simulink model "Joystick_Visualization_2019a"  (R2019a)
settings: Solver=ode1  StartTime=0.0  StopTime=inf  FixedStep=0.001  RelTol=1e-3  EnableMultiTasking=on
undefined symbols (not defined in the file): Host, Visualization
libraries: quarc_library x25, simulink x5
settings Model: SimulationMode=external  ExtModeTrigDuration=10000  Creator=Admin  LastModifiedBy=lgonzalez
settings SolverCC: PositivePriorityOrder=on
settings DataIOCC: SaveFormat=StructureWithTime  ReturnWorkspaceOutputs=off
settings DebuggingCC: SFUnexpectedBacktrackingDiag=warning  SFNoUnconditionalDefaultTransitionDiag=warning  SFExecutionAtInitializationDiag=none  ArithmeticOperatorsInVariantConditions=warning
settings SFSimCC: SimUseLocalCustomCode=off
settings RTWCC: Description=QUARC Win64 Target Using Toolchain  SystemTargetFile=quarc_win64.tlc  TemplateMakefile=quarc_default_tmf  RTWUseLocalCustomCode=off  Toolchain=QUARC win64 | nmake (64-bit Windows)  BuildConfiguration=Faster Runs
settings CodeAppCC: StateflowObjectComments=on
settings STFCustomTargetCC: ConcurrentExecutionCompliant=on  UseToolchainInfoCompliant=on  SystemTargetFile=quarc_win64.tlc
settings GRTTargetCC: TargetLangStandard=C89/C90 (ANSI)  ParMdlRefBuildCompliant=off  CompOptLevelCompliant=off  CombineOutputUpdateFcns=off  MatFileLogging=off  CPPClassGenCompliant=off  GRTInterface=on  ExtMode=on  ExtModeMexFile=quarc_comm
settings ConfigComp: CovMetricSettings=dw  CovSaveCumulativeToWorkspaceVar=on  CovSaveSingleToWorkspaceVar=on  CovExternalEMLEnable=off

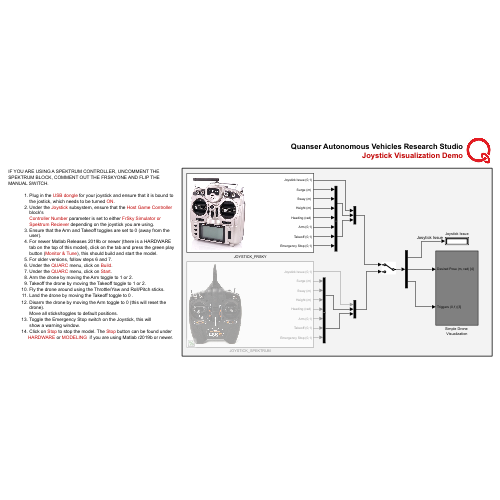
[thumbnail: Simulink's stored preview of the top-level diagram]
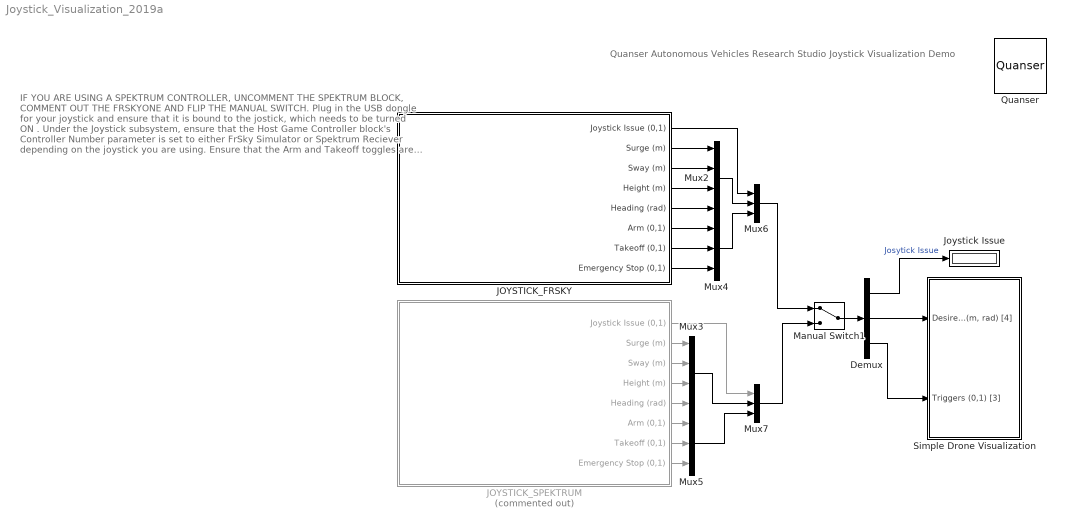
== system Joystick_Visualization_2019a ==
  note: IF YOU ARE USING A SPEKTRUM CONTROLLER, UNCOMMENT THE SPEKTRUM BLOCK, COMMENT OUT THE FRSKYONE AND FLIP THE MANUAL SWITCH.
      |
      | Plug in the USB dongle for your joystick and ensure that it is bound to the jostick, which needs to be turned ON .
      | Under the Joystick subsystem, ensure that the Host Game Controller block's
      | Controller Number parameter is set to either FrSky Simulator or Spektrum Reciever depending on the joystick you are using.
      | Ensure that the Arm and Takeoff toggles are set to 0 (away from the user).
      | For newer Matlab Releases 2019b or newer (there is a HARDWARE tab on the top of this model), click on the tab and press the green play button ( Monitor & Tune ), this should build and start the model.
      | For older versions, follow steps 6 and 7.
      | Under the QUARC menu, click on Build .
      | Under the QUARC menu, click on Start .
      | Arm the drone by moving the Arm toggle to 1 or 2.
      | Takeoff the drone by moving the Takeoff toggle to 1 or 2.
      | Fly the drone around using the Throttle/Yaw and Roll/Pitch sticks.
      | Land the drone by moving the Takeoff toggle to 0 .
      | Disarm the drone by moving the Arm toggle to 0 (this will reset the drone).
      | Move all sticks/toggles to default positions.
      | Toggle the Emergency Stop switch on the Joystick, this will
      | show a warning window.
      | Click on Stop to stop the model. The Stop button can be found under
      | HARDWARE or MODELING if you are using Matlab r2019b or newer.
  note: Quanser Autonomous Vehicles Research Studio
      | Joystick Visualization Demo
  Demux : Demux  Outputs=[1 4 3]
  JOYSTICK_FRSKY : Subsystem
      mask Display: image('frsky.jpg')
  JOYSTICK_SPEKTRUM : Subsystem  Commented=on
      mask Display: image('spektrum.jpg')
  Joystick Issue : Display
      settings: Decimation=400
  Manual Switch1 : ManualSwitch
  Mux2 : Mux
  Mux3 : Mux
  Mux{4..7} (4 alike) : Mux  Inputs=3
  Quanser : quarc_library/Logos/Quanser
  Simple Drone Visualization : Subsystem
  wires:
  Demux/2 -> Simple Drone Visualization/1("Desired Pose (m, rad) [4]")
  Demux/3 -> Simple Drone Visualization/2(Triggers (0,1) [3])
  JOYSTICK_FRSKY/2("Surge (m) ") -> Mux2/1
  JOYSTICK_FRSKY/3("Sway (m) ") -> Mux2/2
  JOYSTICK_FRSKY/4("Height (m) ") -> Mux2/3
  JOYSTICK_FRSKY/5("Heading (rad) ") -> Mux2/4
  JOYSTICK_FRSKY/8(Emergency Stop (0,1)) -> Mux4/3
  JOYSTICK_FRSKY/7(Takeoff (0,1)) -> Mux4/2
  JOYSTICK_FRSKY/6(Arm (0,1)) -> Mux4/1
  JOYSTICK_SPEKTRUM/6(Arm (0,1)) -> Mux5/1
  JOYSTICK_SPEKTRUM/7(Takeoff (0,1)) -> Mux5/2
  JOYSTICK_SPEKTRUM/8(Emergency Stop (0,1)) -> Mux5/3
  JOYSTICK_SPEKTRUM/2("Surge (m) ") -> Mux3/1
  JOYSTICK_SPEKTRUM/3("Sway (m) ") -> Mux3/2
  JOYSTICK_SPEKTRUM/4("Height (m) ") -> Mux3/3
  JOYSTICK_SPEKTRUM/5("Heading (rad) ") -> Mux3/4
  Mux2/1 -> Mux6/2
  Mux4/1 -> Mux6/3
  Mux3/1 -> Mux7/2
  Mux5/1 -> Mux7/3
  Manual Switch1/1 -> Demux/1
  Mux6/1 -> Manual Switch1/1
  Mux7/1 -> Manual Switch1/2
  JOYSTICK_FRSKY/1(Joystick Issue (0,1)) -> Mux6/1
  JOYSTICK_SPEKTRUM/1(Joystick Issue (0,1)) -> Mux7/1
  Demux/1 -> Joystick Issue/1  "Josytick Issue"

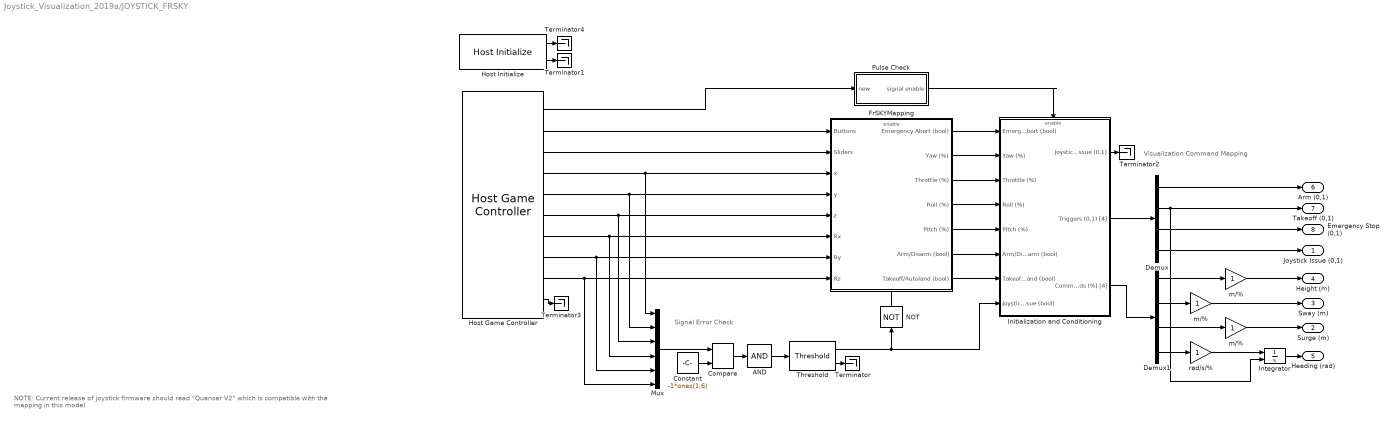
== system Joystick_Visualization_2019a/JOYSTICK_FRSKY ==
  note: NOTE: Current release of joystick firmware should read "Quanser V2" which is compatible with the mapping in this model
  note: Visualization Command Mapping
  note: Signal Error Check
  "  m/%  " : Gain
  " m/% " : Gain
  " rad/s/%" : Gain
  AND : Logic  Inputs=1  AllPortsSameDT=off  OutDataTypeStr=boolean
  Compare : quarc_library/Logic Operations/Compare  operator===  output_data_type=boolean
      settings: SourceProductName=QUARC Targets
  Constant : Constant  Value=-1*ones(1,6)
  Demux : Demux
  Demux1 : Demux
  FrSKYMapping : Subsystem
  Host Game Controller : quarc_library/Devices/Peripherals/Host/Host Game Controller  object_name=Host-1  controller=1  buffer_size=20  deadzone=[]  saturation=[]  sample_time=qc_get_step_size  auto_center=off  enabled=on  debug_mode=off
      settings: SourceProductName=QUARC Targets
  Host Initialize : quarc_library/Devices/Peripherals/Host/Host Initialize  object_name=Host-1  uri_source=Use external mode communications  uri=tcpip://localhost:18001  send_buffer_size=1000  receive_buffer_size=1000  thread_priority=0  run_client=on  use_window=off  window_position=[]  sample_time=qc_get_step_size  active=on
      settings: SourceProductName=QUARC Targets
  Initialization and Conditioning : Subsystem  TreatAsAtomicUnit=on
  Integrator : Integrator  ExternalReset=falling
  Mux : Mux  Inputs=6
  NOT : Logic  Operator=NOT  IconShape=distinctive  AllPortsSameDT=off  OutDataTypeStr=boolean
  Pulse Check : Subsystem  TreatAsAtomicUnit=on
  Terminator{,1..4} (5 alike) : Terminator
  Threshold : quarc_library/Discontinuities/Threshold  operator=>=  param_src=Specify via dialog  threshold=0.5  duration=0.2
      settings: SourceProductName=QUARC Targets
  m/% : Gain
  Joystick Issue (0,1) : Outport  VectorParamsAs1DForOutWhenUnconnected=off
  "Surge (m) " : Outport  Port=2  VectorParamsAs1DForOutWhenUnconnected=off
  "Sway (m) " : Outport  Port=3  VectorParamsAs1DForOutWhenUnconnected=off
  "Height (m) " : Outport  Port=4  VectorParamsAs1DForOutWhenUnconnected=off
  "Heading (rad) " : Outport  Port=5  VectorParamsAs1DForOutWhenUnconnected=off
  Arm (0,1) : Outport  Port=6  VectorParamsAs1DForOutWhenUnconnected=off
  Takeoff (0,1) : Outport  Port=7  VectorParamsAs1DForOutWhenUnconnected=off
  Emergency Stop (0,1) : Outport  Port=8  VectorParamsAs1DForOutWhenUnconnected=off
  wires:
  Host Initialize/1 -> Terminator4/1
  Host Initialize/2 -> Terminator1/1
  Host Game Controller/7 -> Mux/4, FrSKYMapping/6(Rx)
  Constant/1 -> Compare/2
  Threshold/2 -> Terminator/1
  Host Game Controller/10 -> Terminator3/1
  Mux/1 -> Compare/1
  FrSKYMapping/2(Yaw (%)) -> Initialization and Conditioning/2(Yaw (%))
  Host Game Controller/3 -> FrSKYMapping/2(Sliders)
  Host Game Controller/6 -> Mux/3, FrSKYMapping/5(z)
  Initialization and Conditioning/1(Joystick Issue (0,1)) -> Terminator2/1
  " m/% "/1 -> "Sway (m) "/1
  Host Game Controller/9 -> Mux/6, FrSKYMapping/8(Rz)
  FrSKYMapping/3(Throttle (%)) -> Initialization and Conditioning/3(Throttle (%))
  FrSKYMapping/4(Roll (%)) -> Initialization and Conditioning/4(Roll (%))
  Host Game Controller/4 -> Mux/1, FrSKYMapping/3(x)
  Host Game Controller/1 -> Pulse Check/1(new)
  Host Game Controller/5 -> Mux/2, FrSKYMapping/4(y)
  Compare/1 -> AND/1
  FrSKYMapping/7(Takeoff/Autoland (bool)) -> Initialization and Conditioning/7(Takeoff/AutoLand (bool))
  Host Game Controller/2 -> FrSKYMapping/1(Buttons)
  Threshold/1 -> NOT/1, Initialization and Conditioning/8(Joystick Issue (bool))
  Pulse Check/1(signal enable) -> Initialization and Conditioning/Enable
  Initialization and Conditioning/3(Commands (%) [4]) -> Demux1/1
  Demux1/1 -> m/%/1
  FrSKYMapping/1(Emergency Abort (bool)) -> Initialization and Conditioning/1(Emergency Abort (bool))
  Host Game Controller/8 -> Mux/5, FrSKYMapping/7(Ry)
  FrSKYMapping/5(Pitch (%)) -> Initialization and Conditioning/5(Pitch (%))
  m/%/1 -> "Height (m) "/1
  "  m/%  "/1 -> "Surge (m) "/1
  AND/1 -> Threshold/1
  Demux/3 -> Emergency Stop (0,1)/1
  Demux1/2 -> " m/% "/1
  Demux/4 -> Joystick Issue (0,1)/1
  Demux1/4 -> " rad/s/%"/1
  NOT/1 -> FrSKYMapping/Enable
  Demux/2 -> Takeoff (0,1)/1, Integrator/2
  Demux1/3 -> "  m/%  "/1
  FrSKYMapping/6("Arm/Disarm (bool) ") -> Initialization and Conditioning/6(Arm/Disarm (bool))
  Integrator/1 -> "Heading (rad) "/1
  Demux/1 -> Arm (0,1)/1
  " rad/s/%"/1 -> Integrator/1
  Initialization and Conditioning/2(Triggers (0,1) [4]) -> Demux/1

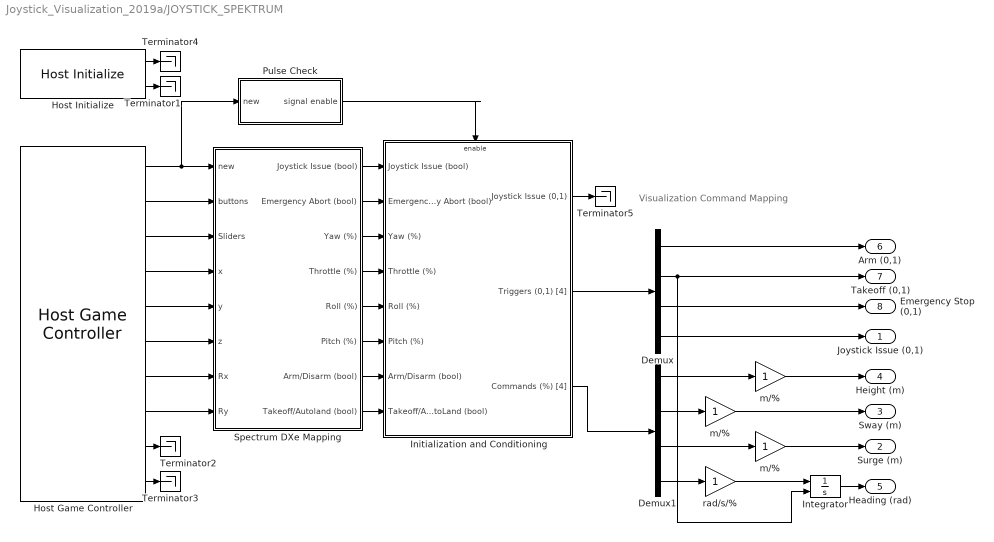
== system Joystick_Visualization_2019a/JOYSTICK_SPEKTRUM ==
  note: Visualization Command Mapping
  "  m/%  " : Gain
  " m/% " : Gain
  " rad/s/%" : Gain
  Demux : Demux
  Demux1 : Demux
  Host Game Controller : quarc_library/Devices/Peripherals/Host/Host Game Controller  object_name=Host-2  controller=1  buffer_size=20  deadzone=[]  saturation=[]  sample_time=qc_get_step_size  auto_center=off  enabled=on  debug_mode=off
      settings: SourceProductName=QUARC Targets
  Host Initialize : quarc_library/Devices/Peripherals/Host/Host Initialize  object_name=Host-2  uri_source=Use external mode communications  uri=tcpip://localhost:18001  send_buffer_size=1000  receive_buffer_size=1000  thread_priority=0  run_client=on  use_window=off  window_position=[]  sample_time=qc_get_step_size  active=on
      settings: SourceProductName=QUARC Targets
  Initialization and Conditioning : Subsystem  TreatAsAtomicUnit=on
  Integrator : Integrator  ExternalReset=falling
  Pulse Check : Subsystem  TreatAsAtomicUnit=on
  Spectrum DXe Mapping : Subsystem
  Terminator{1..5} (5 alike) : Terminator
  m/% : Gain
  Joystick Issue (0,1) : Outport  VectorParamsAs1DForOutWhenUnconnected=off
  "Surge (m) " : Outport  Port=2  VectorParamsAs1DForOutWhenUnconnected=off
  "Sway (m) " : Outport  Port=3  VectorParamsAs1DForOutWhenUnconnected=off
  "Height (m) " : Outport  Port=4  VectorParamsAs1DForOutWhenUnconnected=off
  "Heading (rad) " : Outport  Port=5  VectorParamsAs1DForOutWhenUnconnected=off
  Arm (0,1) : Outport  Port=6  VectorParamsAs1DForOutWhenUnconnected=off
  Takeoff (0,1) : Outport  Port=7  VectorParamsAs1DForOutWhenUnconnected=off
  Emergency Stop (0,1) : Outport  Port=8  VectorParamsAs1DForOutWhenUnconnected=off
  wires:
  Host Game Controller/2 -> Spectrum DXe Mapping/2(buttons)
  Host Initialize/2 -> Terminator1/1
  Host Initialize/1 -> Terminator4/1
  Host Game Controller/6 -> Spectrum DXe Mapping/6(z)
  Host Game Controller/3 -> Spectrum DXe Mapping/3(Sliders)
  Host Game Controller/5 -> Spectrum DXe Mapping/5(y)
  Host Game Controller/4 -> Spectrum DXe Mapping/4(x)
  Host Game Controller/8 -> Spectrum DXe Mapping/8(Ry)
  Host Game Controller/9 -> Terminator2/1
  Host Game Controller/10 -> Terminator3/1
  Host Game Controller/7 -> Spectrum DXe Mapping/7(Rx)
  Demux1/2 -> " m/% "/1
  Spectrum DXe Mapping/2(Emergency Abort (bool)) -> Initialization and Conditioning/2(Emergency Abort (bool))
  Spectrum DXe Mapping/8(Takeoff/Autoland (bool)) -> Initialization and Conditioning/8(Takeoff/AutoLand (bool))
  Demux/1 -> Arm (0,1)/1
  Initialization and Conditioning/3(Commands (%) [4]) -> Demux1/1
  Spectrum DXe Mapping/6(Pitch (%)) -> Initialization and Conditioning/6(Pitch (%))
  Demux/2 -> Takeoff (0,1)/1, Integrator/2
  Integrator/1 -> "Heading (rad) "/1
  Initialization and Conditioning/1(Joystick Issue (0,1)) -> Terminator5/1
  Initialization and Conditioning/2(Triggers (0,1) [4]) -> Demux/1
  Pulse Check/1(signal enable) -> Initialization and Conditioning/Enable
  " rad/s/%"/1 -> Integrator/1
  "  m/%  "/1 -> "Surge (m) "/1
  Spectrum DXe Mapping/4(Throttle (%)) -> Initialization and Conditioning/4(Throttle (%))
  Demux/3 -> Emergency Stop (0,1)/1
  " m/% "/1 -> "Sway (m) "/1
  m/%/1 -> "Height (m) "/1
  Spectrum DXe Mapping/5(Roll (%)) -> Initialization and Conditioning/5(Roll (%))
  Spectrum DXe Mapping/7("Arm/Disarm (bool) ") -> Initialization and Conditioning/7(Arm/Disarm (bool))
  Host Game Controller/1 -> Pulse Check/1(new), Spectrum DXe Mapping/1(new)
  Demux1/1 -> m/%/1
  Spectrum DXe Mapping/3(Yaw (%)) -> Initialization and Conditioning/3(Yaw (%))
  Demux1/3 -> "  m/%  "/1
  Demux1/4 -> " rad/s/%"/1
  Demux/4 -> Joystick Issue (0,1)/1
  Spectrum DXe Mapping/1(Joystick Issue (bool)) -> Initialization and Conditioning/1(Joystick Issue (bool))

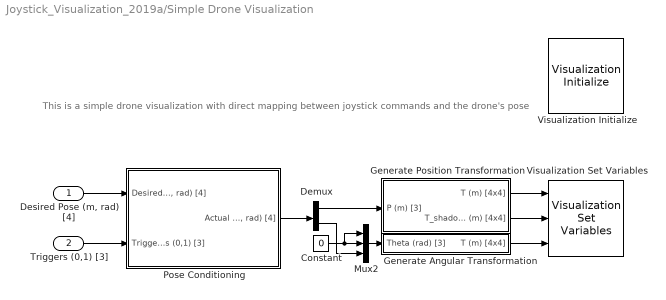
== system Joystick_Visualization_2019a/Simple Drone Visualization ==
  note: This is a simple drone visualization with direct mapping between joystick commands and the drone's pose
  "Desired Pose (m, rad) [4]" : Inport
  Triggers (0,1) [3] : Inport  Port=2
  Constant : Constant  Value=0
  Demux : Demux  Outputs=[3 1]
  Generate Angular Transformation : Subsystem
  Generate Position Transformation : Subsystem
  Mux2 : Mux  Inputs=3
  Pose Conditioning : Subsystem
  Visualization Initialize : quarc_library/User Interface/Visualization/Visualization Initialize  object_name=Visualization-1  scene_file=Quadrotor_Simplified.xml  uri=shmem://%m:2  server_send_size=1000000  server_receive_size=1000  derive_from_server=on  client_send_size=1000  client_receive_size=1000000  variables=[ 33 43 223 ]  initial_values=single([ 1 0 -0 0 0 1 0 0 0 0 1 0 0 0 0 1 1 0 -0 0 0 1 0 0 0 0 1 0 0 0 0 1 1 0 -0 0 0 1 0 0 0 0 1 0 0 0 0 1 ])  open_on_start=on  close_on_stop=on
      settings: AttributesFormatString=%<object_name>  SourceProductName=QUARC Targets
  Visualization Set Variables : quarc_library/User Interface/Visualization/Visualization Set Variables  object_name=Visualization-1  offset=[ 0 32 16 ]  data_type=[ 2 2 2 ]  length=[ 16 16 16 ]  sample_time=visualization_get_frame_period  actor_name={'actor.dummy.Frame.Base/Transform';'actor.dummy.Frame.Shadow/Transform';'actor.dummy.Frame.Body/Transform'}
      settings: AttributesFormatString=(%<object_name>)  SourceProductName=QUARC Targets
  wires:
  Constant/1 -> Mux2/1, Mux2/2
  Mux2/1 -> Generate Angular Transformation/1(Theta (rad) [3])
  Demux/2 -> Mux2/3
  Generate Position Transformation/2(T_shadow (m) [4x4]) -> Visualization Set Variables/2
  Generate Angular Transformation/1(T (m) [4x4]) -> Visualization Set Variables/3
  Generate Position Transformation/1(T (m) [4x4]) -> Visualization Set Variables/1
  Triggers (0,1) [3]/1 -> Pose Conditioning/2(Triggers (0,1) [3])
  "Desired Pose (m, rad) [4]"/1 -> Pose Conditioning/1("Desired Pose (m, rad) [4]")
  Pose Conditioning/1("Actual Pose (m, rad) [4]") -> Demux/1
  Demux/1 -> Generate Position Transformation/1(P (m) [3])

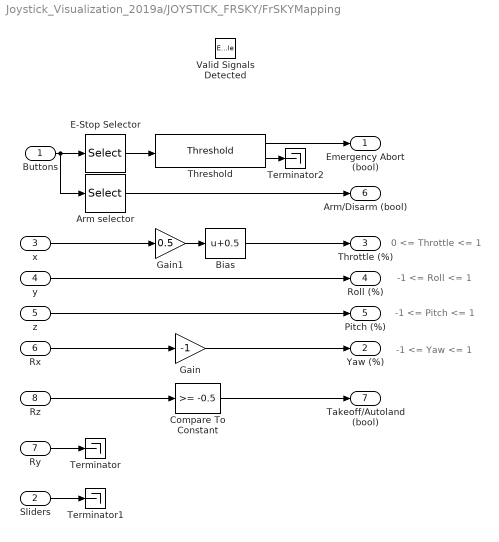
== system Joystick_Visualization_2019a/JOYSTICK_FRSKY/FrSKYMapping ==
  note: -1 <= Yaw <= 1
  note: 0 <= Throttle <= 1
  note: -1 <= Roll <= 1
  note: -1 <= Pitch <= 1
  Buttons : Inport
  Sliders : Inport  Port=2
  x : Inport  Port=3
  y : Inport  Port=4
  z : Inport  Port=5
  Rx : Inport  Port=6
  Ry : Inport  Port=7
  Rz : Inport  Port=8
  Valid Signals Detected : EnablePort
  Arm selector : Selector  InputPortWidth=32  IndexOptions=Index vector (dialog)  Indices=[2]  OutputSizes=1
  Bias : Bias  Bias=0.5
  Compare To Constant : simulink/Logic and Bit Operations/Compare To Constant  relop=>=  const=-0.5  OutDataTypeStr=boolean
  E-Stop Selector : Selector  InputPortWidth=32  IndexOptions=Index vector (dialog)  Indices=[1]  OutputSizes=1
  Gain : Gain  Gain=-1
  Gain1 : Gain  Gain=0.5
  Terminator : Terminator
  Terminator1 : Terminator
  Terminator2 : Terminator
  Threshold : quarc_library/Discontinuities/Threshold  operator=>=  param_src=Specify via dialog  threshold=0.5  duration=0.2
      settings: SourceProductName=QUARC Targets
  Emergency Abort (bool) : Outport  VectorParamsAs1DForOutWhenUnconnected=off
  Yaw (%) : Outport  Port=2  VectorParamsAs1DForOutWhenUnconnected=off
  Throttle (%) : Outport  Port=3  VectorParamsAs1DForOutWhenUnconnected=off
  Roll (%) : Outport  Port=4  VectorParamsAs1DForOutWhenUnconnected=off
  Pitch (%) : Outport  Port=5  VectorParamsAs1DForOutWhenUnconnected=off
  "Arm/Disarm (bool) " : Outport  Port=6  VectorParamsAs1DForOutWhenUnconnected=off
  Takeoff/Autoland (bool) : Outport  Port=7  VectorParamsAs1DForOutWhenUnconnected=off
  wires:
  Buttons/1 -> Arm selector/1, E-Stop Selector/1
  Arm selector/1 -> "Arm/Disarm (bool) "/1
  x/1 -> Gain1/1
  y/1 -> Roll (%)/1
  z/1 -> Pitch (%)/1
  Rx/1 -> Gain/1
  Ry/1 -> Terminator/1
  Sliders/1 -> Terminator1/1
  E-Stop Selector/1 -> Threshold/1
  Rz/1 -> Compare To Constant/1
  Compare To Constant/1 -> Takeoff/Autoland (bool)/1
  Threshold/1 -> Emergency Abort (bool)/1
  Threshold/2 -> Terminator2/1
  Gain/1 -> Yaw (%)/1
  Gain1/1 -> Bias/1
  Bias/1 -> Throttle (%)/1

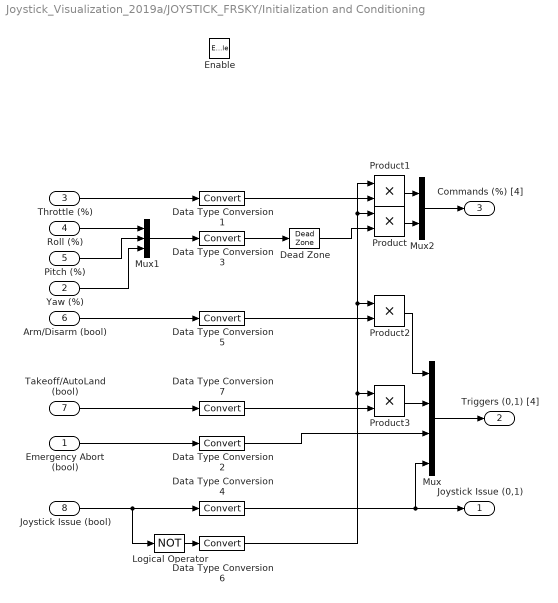
== system Joystick_Visualization_2019a/JOYSTICK_FRSKY/Initialization and Conditioning ==
  Emergency Abort (bool) : Inport
  Yaw (%) : Inport  Port=2
  Throttle (%) : Inport  Port=3
  Roll (%) : Inport  Port=4
  Pitch (%) : Inport  Port=5
  Arm/Disarm (bool) : Inport  Port=6
  Takeoff/AutoLand (bool) : Inport  Port=7
  Joystick Issue (bool) : Inport  Port=8
  Enable : EnablePort  StatesWhenEnabling=reset
  Data Type Conversion{1..7} (7 alike) : DataTypeConversion
  Dead Zone : DeadZone  LowerValue=-0.01  UpperValue=0.01  SaturateOnIntegerOverflow=on
  Logical Operator : Logic  Operator=NOT  AllPortsSameDT=off  OutDataTypeStr=boolean
  Mux : Mux
  Mux1 : Mux  Inputs=3
  Mux2 : Mux  Inputs=2
  Product{,1..3} (4 alike) : Product
  Joystick Issue (0,1) : Outport  InitialOutput=0  VectorParamsAs1DForOutWhenUnconnected=off
  Triggers (0,1) [4] : Outport  Port=2  InitialOutput=0  VectorParamsAs1DForOutWhenUnconnected=off
  Commands (%) [4] : Outport  Port=3  InitialOutput=0  VectorParamsAs1DForOutWhenUnconnected=off
  wires:
  Joystick Issue (bool)/1 -> Data Type Conversion4/1, Logical Operator/1
  Mux1/1 -> Data Type Conversion3/1
  Throttle (%)/1 -> Data Type Conversion1/1
  Roll (%)/1 -> Mux1/1
  Pitch (%)/1 -> Mux1/2
  Yaw (%)/1 -> Mux1/3
  Data Type Conversion4/1 -> Mux/4, Joystick Issue (0,1)/1
  Emergency Abort (bool)/1 -> Data Type Conversion2/1
  Data Type Conversion3/1 -> Dead Zone/1
  Arm/Disarm (bool)/1 -> Data Type Conversion5/1
  Mux/1 -> Triggers (0,1) [4]/1
  Data Type Conversion2/1 -> Mux/3
  Logical Operator/1 -> Data Type Conversion6/1
  Product/1 -> Mux2/2
  Product1/1 -> Mux2/1
  Data Type Conversion1/1 -> Product1/2
  Dead Zone/1 -> Product/2
  Data Type Conversion6/1 -> Product1/1, Product/1, Product2/1, Product3/1
  Product2/1 -> Mux/1
  Data Type Conversion5/1 -> Product2/2
  Takeoff/AutoLand (bool)/1 -> Data Type Conversion7/1
  Product3/1 -> Mux/2
  Data Type Conversion7/1 -> Product3/2
  Mux2/1 -> Commands (%) [4]/1

== system Joystick_Visualization_2019a/JOYSTICK_FRSKY/Pulse Check ==
  note: For this subsystem we will count the number of new pulses. The data can be considered enabled once the count of new signals has gone beyond 1. This will enable the Initializing and conditioning subsystem.
  new : Inport
  Compare : quarc_library/Logic Operations/Compare  operator=>=  output_data_type=boolean
      settings: SourceProductName=QUARC Targets
  Pulse Check : Constant
  "pulse count " : Subsystem  TreatAsAtomicUnit=on
  signal enable : Outport  InitialOutput=0  VectorParamsAs1DForOutWhenUnconnected=off
  wires:
  Compare/1 -> signal enable/1
  Pulse Check/1 -> Compare/2
  new/1 -> "pulse count "/Trigger
  "pulse count "/1(Number of Pulses) -> Compare/1

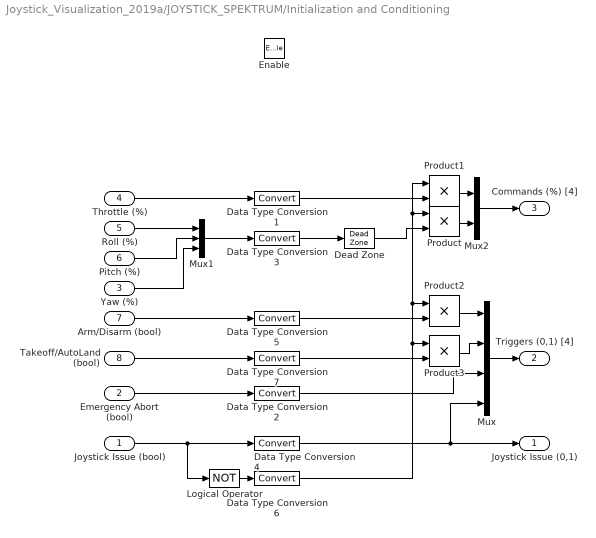
== system Joystick_Visualization_2019a/JOYSTICK_SPEKTRUM/Initialization and Conditioning ==
  Joystick Issue (bool) : Inport
  Emergency Abort (bool) : Inport  Port=2
  Yaw (%) : Inport  Port=3
  Throttle (%) : Inport  Port=4
  Roll (%) : Inport  Port=5
  Pitch (%) : Inport  Port=6
  Arm/Disarm (bool) : Inport  Port=7
  Takeoff/AutoLand (bool) : Inport  Port=8
  Enable : EnablePort  StatesWhenEnabling=reset
  Data Type Conversion{1..7} (7 alike) : DataTypeConversion
  Dead Zone : DeadZone  LowerValue=-0.01  UpperValue=0.01  SaturateOnIntegerOverflow=on
  Logical Operator : Logic  Operator=NOT  AllPortsSameDT=off  OutDataTypeStr=boolean
  Mux : Mux
  Mux1 : Mux  Inputs=3
  Mux2 : Mux  Inputs=2
  Product{,1..3} (4 alike) : Product
  Joystick Issue (0,1) : Outport  InitialOutput=0  VectorParamsAs1DForOutWhenUnconnected=off
  Triggers (0,1) [4] : Outport  Port=2  InitialOutput=0  VectorParamsAs1DForOutWhenUnconnected=off
  Commands (%) [4] : Outport  Port=3  InitialOutput=0  VectorParamsAs1DForOutWhenUnconnected=off
  wires:
  Joystick Issue (bool)/1 -> Data Type Conversion4/1, Logical Operator/1
  Mux1/1 -> Data Type Conversion3/1
  Throttle (%)/1 -> Data Type Conversion1/1
  Roll (%)/1 -> Mux1/1
  Pitch (%)/1 -> Mux1/2
  Yaw (%)/1 -> Mux1/3
  Data Type Conversion4/1 -> Mux/4, Joystick Issue (0,1)/1
  Emergency Abort (bool)/1 -> Data Type Conversion2/1
  Data Type Conversion3/1 -> Dead Zone/1
  Arm/Disarm (bool)/1 -> Data Type Conversion5/1
  Mux/1 -> Triggers (0,1) [4]/1
  Data Type Conversion2/1 -> Mux/3
  Logical Operator/1 -> Data Type Conversion6/1
  Product/1 -> Mux2/2
  Product1/1 -> Mux2/1
  Data Type Conversion1/1 -> Product1/2
  Dead Zone/1 -> Product/2
  Data Type Conversion6/1 -> Product1/1, Product/1, Product2/1, Product3/1
  Product2/1 -> Mux/1
  Data Type Conversion5/1 -> Product2/2
  Takeoff/AutoLand (bool)/1 -> Data Type Conversion7/1
  Product3/1 -> Mux/2
  Data Type Conversion7/1 -> Product3/2
  Mux2/1 -> Commands (%) [4]/1

== system Joystick_Visualization_2019a/JOYSTICK_SPEKTRUM/Pulse Check ==
  note: For this subsystem we will count the number of new pulses. The data can be considered enabled once the count of new signals has gone beyond 2. This will enable the Initializing and conditioning subsystem.
  new : Inport
  Compare : quarc_library/Logic Operations/Compare  operator=>  output_data_type=boolean
      settings: SourceProductName=QUARC Targets
  Pulse Check : Constant  Value=2
  "pulse count " : Subsystem  TreatAsAtomicUnit=on
  signal enable : Outport  InitialOutput=0  VectorParamsAs1DForOutWhenUnconnected=off
  wires:
  "pulse count "/1(Number of Pulses) -> Compare/1
  new/1 -> "pulse count "/Trigger
  Pulse Check/1 -> Compare/2
  Compare/1 -> signal enable/1

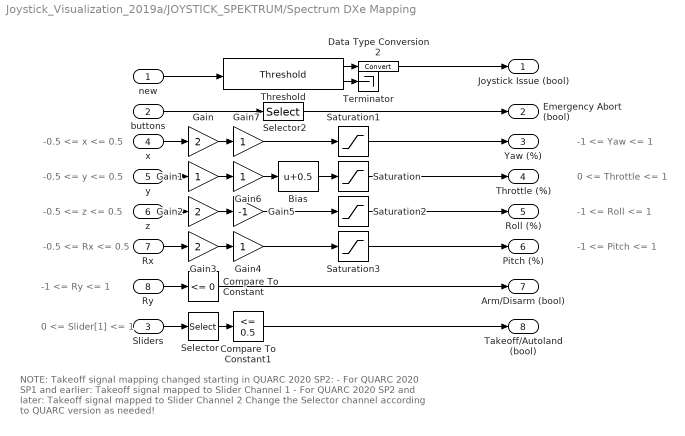
== system Joystick_Visualization_2019a/JOYSTICK_SPEKTRUM/Spectrum DXe Mapping ==
  note: NOTE: Takeoff signal mapping changed starting in QUARC 2020 SP2:
      |
      | - For QUARC 2020 SP1 and earlier: Takeoff signal mapped to Slider Channel 1
      | - For QUARC 2020 SP2 and later: Takeoff signal mapped to Slider Channel 2
      |
      | Change the Selector channel according to QUARC version as needed!
  note: -1 <= Ry <= 1
  note: 0 <= Slider[1] <= 1
  note: -1 <= Pitch <= 1
  note: -0.5 <= Rx <= 0.5
  note: -1 <= Roll <= 1
  note: -0.5 <= z <= 0.5
  note: 0 <= Throttle <= 1
  note: -0.5 <= y <= 0.5
  note: -1 <= Yaw <= 1
  note: -0.5 <= x <= 0.5
  new : Inport
  buttons : Inport  Port=2
  Sliders : Inport  Port=3
  x : Inport  Port=4
  y : Inport  Port=5
  z : Inport  Port=6
  Rx : Inport  Port=7
  Ry : Inport  Port=8
  Bias : Bias  Bias=0.5
  Compare To Constant : simulink/Logic and Bit Operations/Compare To Constant  relop=<=  const=0  OutDataTypeStr=boolean
  Compare To Constant1 : simulink/Logic and Bit Operations/Compare To Constant  relop=<=  const=0.5  OutDataTypeStr=boolean
  Data Type Conversion2 : DataTypeConversion
  Gain : Gain  Gain=2
  Gain{1,4,6..7} (4 alike) : Gain
  Gain2 : Gain  Gain=2
  Gain3 : Gain  Gain=2
  Gain5 : Gain  Gain=-1
  Saturation : Saturate  UpperLimit=1  LowerLimit=0
  Saturation1 : Saturate  UpperLimit=1  LowerLimit=-1
  Saturation2 : Saturate  UpperLimit=1  LowerLimit=-1
  Saturation3 : Saturate  UpperLimit=1  LowerLimit=-1
  Selector : Selector  InputPortWidth=2  IndexOptions=Index vector (dialog)  Indices=[2]  OutputSizes=1
  Selector2 : Selector  InputPortWidth=32  IndexOptions=Index vector (dialog)  Indices=[1]  OutputSizes=1
  Terminator : Terminator
  Threshold : quarc_library/Discontinuities/Threshold  operator===  param_src=Specify via dialog  threshold=0  duration=1
      settings: SourceProductName=QUARC Targets
  Joystick Issue (bool) : Outport  VectorParamsAs1DForOutWhenUnconnected=off
  Emergency Abort (bool) : Outport  Port=2  VectorParamsAs1DForOutWhenUnconnected=off
  Yaw (%) : Outport  Port=3  VectorParamsAs1DForOutWhenUnconnected=off
  Throttle (%) : Outport  Port=4  VectorParamsAs1DForOutWhenUnconnected=off
  Roll (%) : Outport  Port=5  VectorParamsAs1DForOutWhenUnconnected=off
  Pitch (%) : Outport  Port=6  VectorParamsAs1DForOutWhenUnconnected=off
  "Arm/Disarm (bool) " : Outport  Port=7  VectorParamsAs1DForOutWhenUnconnected=off
  Takeoff/Autoland (bool) : Outport  Port=8  VectorParamsAs1DForOutWhenUnconnected=off
  wires:
  Data Type Conversion2/1 -> Joystick Issue (bool)/1
  new/1 -> Threshold/1
  Threshold/1 -> Data Type Conversion2/1
  Selector2/1 -> Emergency Abort (bool)/1
  Threshold/2 -> Terminator/1
  buttons/1 -> Selector2/1
  Compare To Constant1/1 -> Takeoff/Autoland (bool)/1
  Rx/1 -> Gain3/1
  y/1 -> Gain1/1
  Ry/1 -> Compare To Constant/1
  x/1 -> Gain/1
  z/1 -> Gain2/1
  Gain4/1 -> Saturation3/1
  Gain1/1 -> Gain6/1
  Gain2/1 -> Gain5/1
  Bias/1 -> Saturation/1
  Saturation2/1 -> Roll (%)/1
  Gain3/1 -> Gain4/1
  Gain/1 -> Gain7/1
  Saturation1/1 -> Yaw (%)/1
  Gain6/1 -> Bias/1
  Sliders/1 -> Selector/1
  Saturation/1 -> Throttle (%)/1
  Gain5/1 -> Saturation2/1
  Selector/1 -> Compare To Constant1/1
  Gain7/1 -> Saturation1/1
  Saturation3/1 -> Pitch (%)/1
  Compare To Constant/1 -> "Arm/Disarm (bool) "/1

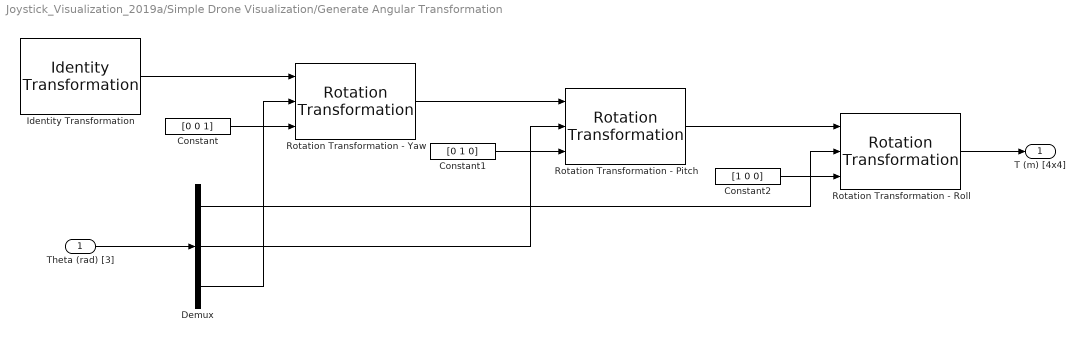
== system Joystick_Visualization_2019a/Simple Drone Visualization/Generate Angular Transformation ==
  Theta (rad) [3] : Inport
  Constant : Constant  Value=[0 0 1]
  Constant1 : Constant  Value=[0 1 0]
  Constant2 : Constant  Value=[1 0 0]
  Demux : Demux  Outputs=3
  Identity Transformation : quarc_library/Math Operations/Homogeneous Transformations/Identity  Transformation
      settings: SourceProductName=QUARC Targets
  Rotation Transformation - Pitch : quarc_library/Math Operations/Homogeneous Transformations/Rotation Transformation  angle_source=Use external input  angle=0  axis_source=Use external input  axis=[0 0 1]
      settings: SourceProductName=QUARC Targets
  Rotation Transformation - Roll : quarc_library/Math Operations/Homogeneous Transformations/Rotation Transformation  angle_source=Use external input  angle=0  axis_source=Use external input  axis=[0 0 1]
      settings: SourceProductName=QUARC Targets
  Rotation Transformation - Yaw : quarc_library/Math Operations/Homogeneous Transformations/Rotation Transformation  angle_source=Use external input  angle=0  axis_source=Use external input  axis=[0 0 1]
      settings: SourceProductName=QUARC Targets
  T (m) [4x4] : Outport  VectorParamsAs1DForOutWhenUnconnected=off
  wires:
  Rotation Transformation - Roll/1 -> T (m) [4x4]/1
  Identity Transformation/1 -> Rotation Transformation - Yaw/1
  Constant/1 -> Rotation Transformation - Yaw/3
  Rotation Transformation - Yaw/1 -> Rotation Transformation - Pitch/1
  Constant1/1 -> Rotation Transformation - Pitch/3
  Constant2/1 -> Rotation Transformation - Roll/3
  Rotation Transformation - Pitch/1 -> Rotation Transformation - Roll/1
  Demux/1 -> Rotation Transformation - Roll/2
  Theta (rad) [3]/1 -> Demux/1
  Demux/3 -> Rotation Transformation - Yaw/2
  Demux/2 -> Rotation Transformation - Pitch/2

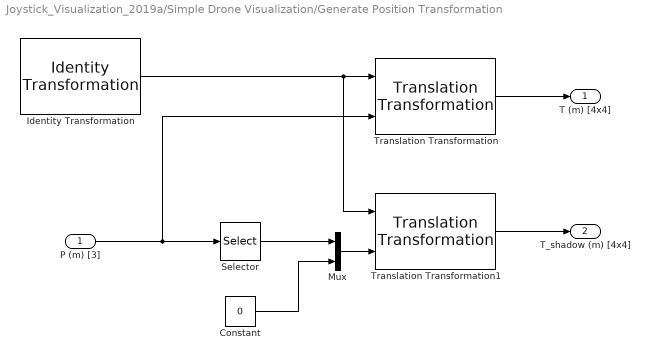
== system Joystick_Visualization_2019a/Simple Drone Visualization/Generate Position Transformation ==
  P (m) [3] : Inport
  Constant : Constant  Value=0
  Identity Transformation : quarc_library/Math Operations/Homogeneous Transformations/Identity  Transformation
      settings: SourceProductName=QUARC Targets
  Mux : Mux  Inputs=2
  Selector : Selector  InputPortWidth=3  IndexOptions=Index vector (dialog)  Indices=[1 2]  OutputSizes=1
  Translation Transformation : quarc_library/Math Operations/Homogeneous Transformations/Translation Transformation  source=Use external input  translation=[0 0 0]
      settings: SourceProductName=QUARC Targets
  Translation Transformation1 : quarc_library/Math Operations/Homogeneous Transformations/Translation Transformation  source=Use external input  translation=[0 0 0]
      settings: SourceProductName=QUARC Targets
  T (m) [4x4] : Outport  VectorParamsAs1DForOutWhenUnconnected=off
  T_shadow (m) [4x4] : Outport  Port=2  VectorParamsAs1DForOutWhenUnconnected=off
  wires:
  Identity Transformation/1 -> Translation Transformation1/1, Translation Transformation/1
  Translation Transformation/1 -> T (m) [4x4]/1
  P (m) [3]/1 -> Translation Transformation/2, Selector/1
  Selector/1 -> Mux/1
  Mux/1 -> Translation Transformation1/2
  Constant/1 -> Mux/2
  Translation Transformation1/1 -> T_shadow (m) [4x4]/1

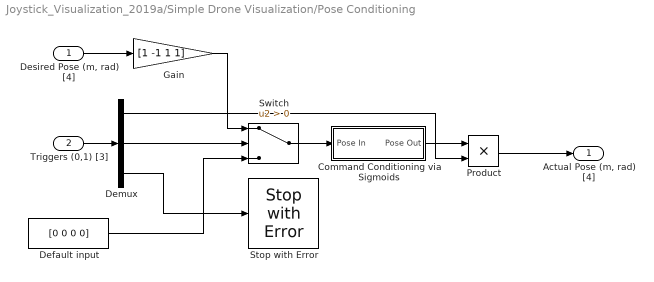
== system Joystick_Visualization_2019a/Simple Drone Visualization/Pose Conditioning ==
  "Desired Pose (m, rad) [4]" : Inport
  Triggers (0,1) [3] : Inport  Port=2
  Command Conditioning via Sigmoids : Subsystem
  "Default input " : Constant  Value=[0 0 0 0]
  Demux : Demux  Outputs=3
  Gain : Gain  Gain=[1 -1 1 1]
  Product : Product
  Stop with Error : quarc_library/Sinks/Error Handling/Stop with Error  message_type=Fixed error message  message=E-Stop Toggled!
      settings: AttributesFormatString="\"%<message>\""  SourceProductName=QUARC Targets
  Switch : Switch  Criteria=u2 > Threshold
  "Actual Pose (m, rad) [4]" : Outport  VectorParamsAs1DForOutWhenUnconnected=off
  wires:
  "Desired Pose (m, rad) [4]"/1 -> Gain/1
  Triggers (0,1) [3]/1 -> Demux/1
  Product/1 -> "Actual Pose (m, rad) [4]"/1
  Demux/1 -> Product/2
  Command Conditioning via Sigmoids/1(Pose Out) -> Product/1
  Demux/2 -> Switch/2
  Gain/1 -> Switch/1
  "Default input "/1 -> Switch/3
  Switch/1 -> Command Conditioning via Sigmoids/1(Pose In)
  Demux/3 -> Stop with Error/1

== system Joystick_Visualization_2019a/JOYSTICK_FRSKY/Pulse Check/pulse count  ==
  Trigger : TriggerPort  TriggerType=either  VariantControl=Variant
  Constant1 : Constant  Value=0
  Increment Stored Integer : simulink/Additional Math & Discrete/Additional Math: Increment - Decrement/Increment Stored Integer
  Sum : Sum  Inputs=|++
  Unit Delay : UnitDelay  SampleTime=-1  HasFrameUpgradeWarning=on
  Number of Pulses : Outport  VectorParamsAs1DForOutWhenUnconnected=off
  wires:
  Constant1/1 -> Sum/1
  Sum/1 -> Increment Stored Integer/1
  Unit Delay/1 -> Sum/2
  Increment Stored Integer/1 -> Unit Delay/1, Number of Pulses/1

== system Joystick_Visualization_2019a/JOYSTICK_SPEKTRUM/Pulse Check/pulse count  ==
  Trigger : TriggerPort  VariantControl=Variant
  Constant1 : Constant  Value=0
  Increment Stored Integer : simulink/Additional Math & Discrete/Additional Math: Increment - Decrement/Increment Stored Integer
  Sum : Sum  Inputs=|++
  Unit Delay : UnitDelay  SampleTime=-1  HasFrameUpgradeWarning=on
  Number of Pulses : Outport  VectorParamsAs1DForOutWhenUnconnected=off
  wires:
  Increment Stored Integer/1 -> Number of Pulses/1, Unit Delay/1
  Unit Delay/1 -> Sum/2
  Sum/1 -> Increment Stored Integer/1
  Constant1/1 -> Sum/1

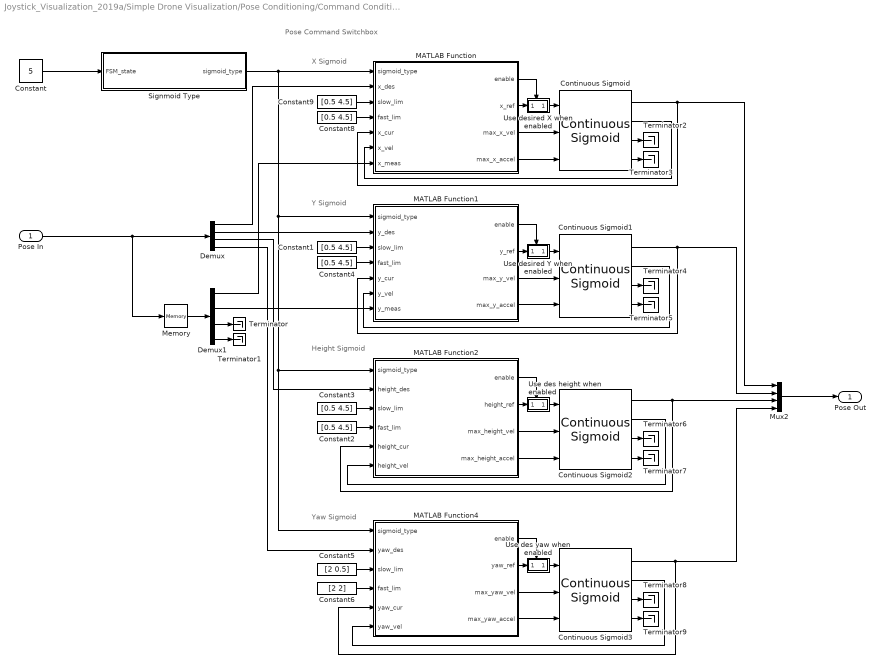
== system Joystick_Visualization_2019a/Simple Drone Visualization/Pose Conditioning/Command Conditioning via Sigmoids ==
  note: Pose Command Switchbox
  note: X Sigmoid
  note: Y Sigmoid
  note: Height Sigmoid
  note: Yaw Sigmoid
  Pose In : Inport
  Constant : Constant  Value=5
  Constant{1..4,8..9} (6 alike) : Constant  Value=[0.5 4.5]
  Constant5 : Constant  Value=[2 0.5]
  Constant6 : Constant  Value=[2 2]
  Continuous Sigmoid{,1..3} (4 alike) : quarc_library/Sources/Sigmoids/Continuous Sigmoid  params_source=External (input ports)  max_velocity=2  max_acceleration=10  initial_position=0  initial_velocity=0  hold_off=0.5  input_sample_time=-1  output_sample_time=qc_get_step_size
      settings: SourceProductName=QUARC Targets
  Demux : Demux
  Demux1 : Demux
  MATLAB Function : MATLAB Function  TreatAsAtomicUnit=on
  MATLAB Function1 : MATLAB Function  TreatAsAtomicUnit=on
  MATLAB Function2 : MATLAB Function  TreatAsAtomicUnit=on
  MATLAB Function4 : MATLAB Function  TreatAsAtomicUnit=on
  Memory : Memory
  Mux2 : Mux
  Signmoid Type : MATLAB Function  TreatAsAtomicUnit=on
  Terminator{,1..9} (10 alike) : Terminator
  Use des height when enabled : Subsystem  TreatAsAtomicUnit=on
  Use des yaw when enabled : Subsystem  TreatAsAtomicUnit=on
  Use desired X when enabled : Subsystem  TreatAsAtomicUnit=on
  Use desired Y when enabled : Subsystem  TreatAsAtomicUnit=on
  Pose Out : Outport  VectorParamsAs1DForOutWhenUnconnected=off
  wires:
  MATLAB Function4/2(yaw_ref) -> Use des yaw when enabled/1(h_d (m) [1])
  Demux/2 -> MATLAB Function1/2(y_des)
  MATLAB Function4/3(max_yaw_vel) -> Continuous Sigmoid3/2
  Demux/1 -> MATLAB Function/2(x_des)
  Constant5/1 -> MATLAB Function4/3(slow_lim)
  Constant2/1 -> MATLAB Function2/4(fast_lim)
  Continuous Sigmoid2/1 -> MATLAB Function2/5(height_cur), Mux2/3
  Continuous Sigmoid/1 -> MATLAB Function/5(x_cur), Mux2/1
  Continuous Sigmoid/4 -> Terminator3/1
  MATLAB Function/3(max_x_vel) -> Continuous Sigmoid/2
  Continuous Sigmoid2/3 -> Terminator6/1
  MATLAB Function2/4(max_height_accel) -> Continuous Sigmoid2/3
  MATLAB Function2/1(enable) -> Use des height when enabled/Enable
  MATLAB Function/4(max_x_accel) -> Continuous Sigmoid/3
  Demux1/2 -> MATLAB Function1/7(y_meas)
  Continuous Sigmoid/3 -> Terminator2/1
  Continuous Sigmoid3/2 -> MATLAB Function4/6(yaw_vel)
  MATLAB Function2/2(height_ref) -> Use des height when enabled/1(h_d (m) [1])
  Continuous Sigmoid/2 -> MATLAB Function/6(x_vel)
  MATLAB Function/1(enable) -> Use desired X when enabled/Enable
  Demux/4 -> MATLAB Function4/2(yaw_des)
  MATLAB Function4/1(enable) -> Use des yaw when enabled/Enable
  Use des height when enabled/1(Out1) -> Continuous Sigmoid2/1
  MATLAB Function1/3(max_y_vel) -> Continuous Sigmoid1/2
  MATLAB Function2/3(max_height_vel) -> Continuous Sigmoid2/2
  Continuous Sigmoid1/3 -> Terminator4/1
  Constant8/1 -> MATLAB Function/4(fast_lim)
  Continuous Sigmoid3/1 -> MATLAB Function4/5(yaw_cur), Mux2/4
  MATLAB Function1/4(max_y_accel) -> Continuous Sigmoid1/3
  Continuous Sigmoid2/2 -> MATLAB Function2/6(height_vel)
  Continuous Sigmoid2/4 -> Terminator7/1
  Constant9/1 -> MATLAB Function/3(slow_lim)
  MATLAB Function4/4(max_yaw_accel) -> Continuous Sigmoid3/3
  Demux1/3 -> Terminator/1
  Demux/3 -> MATLAB Function2/2(height_des)
  MATLAB Function1/1(enable) -> Use desired Y when enabled/Enable
  Signmoid Type/1(sigmoid_type) -> MATLAB Function4/1(sigmoid_type), MATLAB Function2/1(sigmoid_type), MATLAB Function1/1(sigmoid_type), MATLAB Function/1(sigmoid_type)
  Mux2/1 -> Pose Out/1
  MATLAB Function1/2(y_ref) -> Use desired Y when enabled/1(h_d (m) [1])
  Demux1/1 -> MATLAB Function/7(x_meas)
  Constant6/1 -> MATLAB Function4/4(fast_lim)
  Use des yaw when enabled/1(Out1) -> Continuous Sigmoid3/1
  Constant4/1 -> MATLAB Function1/4(fast_lim)
  Constant3/1 -> MATLAB Function2/3(slow_lim)
  Use desired Y when enabled/1(Out1) -> Continuous Sigmoid1/1
  Continuous Sigmoid3/4 -> Terminator9/1
  Constant1/1 -> MATLAB Function1/3(slow_lim)
  Continuous Sigmoid1/4 -> Terminator5/1
  Continuous Sigmoid1/2 -> MATLAB Function1/6(y_vel)
  MATLAB Function/2(x_ref) -> Use desired X when enabled/1(h_d (m) [1])
  Demux1/4 -> Terminator1/1
  Continuous Sigmoid3/3 -> Terminator8/1
  Continuous Sigmoid1/1 -> MATLAB Function1/5(y_cur), Mux2/2
  Use desired X when enabled/1(Out1) -> Continuous Sigmoid/1
  Pose In/1 -> Demux/1, Memory/1
  Constant/1 -> Signmoid Type/1(FSM_state)
  Memory/1 -> Demux1/1

== system Joystick_Visualization_2019a/Simple Drone Visualization/Pose Conditioning/Command Conditioning via Sigmoids/Use des height when enabled ==
  h_d (m) [1] : Inport
  Enable : EnablePort
  Out1 : Outport  OutputWhenDisabled=reset  InitialOutput=0  VectorParamsAs1DForOutWhenUnconnected=off
  wires:
  h_d (m) [1]/1 -> Out1/1

== system Joystick_Visualization_2019a/Simple Drone Visualization/Pose Conditioning/Command Conditioning via Sigmoids/Use des yaw when enabled ==
  h_d (m) [1] : Inport
  Enable : EnablePort
  Out1 : Outport  OutputWhenDisabled=reset  InitialOutput=0  VectorParamsAs1DForOutWhenUnconnected=off
  wires:
  h_d (m) [1]/1 -> Out1/1

== system Joystick_Visualization_2019a/Simple Drone Visualization/Pose Conditioning/Command Conditioning via Sigmoids/Use desired X when enabled ==
  h_d (m) [1] : Inport
  Enable : EnablePort
  Out1 : Outport  OutputWhenDisabled=reset  InitialOutput=0  VectorParamsAs1DForOutWhenUnconnected=off
  wires:
  h_d (m) [1]/1 -> Out1/1

== system Joystick_Visualization_2019a/Simple Drone Visualization/Pose Conditioning/Command Conditioning via Sigmoids/Use desired Y when enabled ==
  h_d (m) [1] : Inport
  Enable : EnablePort
  Out1 : Outport  OutputWhenDisabled=reset  InitialOutput=0  VectorParamsAs1DForOutWhenUnconnected=off
  wires:
  h_d (m) [1]/1 -> Out1/1

== matlab function Joystick_Visualization_2019a/Simple Drone Visualization/Pose Conditioning/Command Conditioning via Sigmoids/MATLAB Function ==
  data: sigmoid_type input; enable output; x_des input; slow_lim input; fast_lim input; x_cur input; x_vel input; x_ref output; max_x_vel output; max_x_accel output; x_meas input
function [enable, x_ref, max_x_vel, max_x_accel] = fcn(sigmoid_type, x_des, slow_lim, fast_lim, x_cur, x_vel, x_meas)
%#codegen

enable = 0;
x_ref = 0;
max_x_vel = 0;
max_x_accel = 0;

switch sigmoid_type
    case 1 % Do not pass in x reference
        enable = 1;
        x_ref = x_meas;
        max_x_vel = slow_lim(1);
        max_x_accel = slow_lim(2);

    case 2 % This is different from Case 1 in the measurement selection
        enable = 1;
        x_ref = x_meas;
        max_x_vel = slow_lim(1);
        max_x_accel = slow_lim(2);

    case 3 % 
        enable = 1;
        x_ref = x_des;
        max_x_vel = fast_lim(1);
        max_x_accel = fast_lim(2);

    case 4
        enable = 1;
        x_ref = x_des;
        if (abs(x_cur - x_des) <= 0.02)
            max_x_vel = fast_lim(1);
            max_x_accel = fast_lim(2);
        else    
            max_x_vel = slow_lim(1);
            max_x_accel = slow_lim(2);
        end
    case 5
        enable = 1;
        x_ref = x_des;
        if (abs(x_cur - x_des) <= 0.02)
            max_x_vel = fast_lim(1);
            max_x_accel = fast_lim(2);        
        else
            max_x_vel = slow_lim(1);
            max_x_accel = slow_lim(2);
        end
        
end

== matlab function Joystick_Visualization_2019a/Simple Drone Visualization/Pose Conditioning/Command Conditioning via Sigmoids/MATLAB Function1 ==
  data: sigmoid_type input; enable output; y_des input; slow_lim input; fast_lim input; y_cur input; y_vel input; y_ref output; max_y_vel output; max_y_accel output; y_meas input
function [enable, y_ref, max_y_vel, max_y_accel] = fcn(sigmoid_type, y_des, slow_lim, fast_lim, y_cur, y_vel, y_meas)
%#codegen

enable = 0;
y_ref = 0;
max_y_vel = 0;
max_y_accel = 0;

switch sigmoid_type
    case 1 % Do not pass in x reference
        enable = 1;
        y_ref = y_meas;
        max_y_vel = slow_lim(1);
        max_y_accel = slow_lim(2);

    case 2 % This is different from Case 1 in the measurement selection
        enable = 1;
        y_ref = y_meas;
        max_y_vel = slow_lim(1);
        max_y_accel = slow_lim(2);

    case 3 % 
        enable = 1;
        y_ref = y_des;
        max_y_vel = fast_lim(1);
        max_y_accel = fast_lim(2);

    case 4
        enable = 1;
        y_ref = y_des;
        if (abs(y_cur - y_des) <= 0.02)
            max_y_vel = fast_lim(1);
            max_y_accel = fast_lim(2);
        else    
            max_y_vel = slow_lim(1);
            max_y_accel = slow_lim(2);
        end
    case 5
        enable = 1;
        y_ref = y_des;
        if (abs(y_cur - y_des) <= 0.02)
            max_y_vel = fast_lim(1);
            max_y_accel = fast_lim(2);        
        else
            max_y_vel = slow_lim(1);
            max_y_accel = slow_lim(2);
        end
        
end

== matlab function Joystick_Visualization_2019a/Simple Drone Visualization/Pose Conditioning/Command Conditioning via Sigmoids/MATLAB Function2 ==
  data: sigmoid_type input; enable output; height_des input; slow_lim input; fast_lim input; height_cur input; height_vel input; height_ref output; max_height_vel output; max_height_accel output
function [enable, height_ref, max_height_vel, max_height_accel] = fcn(sigmoid_type, height_des, slow_lim, fast_lim, height_cur, height_vel)
%#codegen

enable = 0;
height_ref = 0;
max_height_vel = 0;
max_height_accel = 0;

switch sigmoid_type
    case 1 % Do not pass in height reference
        enable = 0;
        height_ref = 0;
        max_height_vel = 0;
        max_height_accel = 0;

    case 2 % This is different from Case 1 in the measurement selection
        enable = 0;
        height_ref = 0;
        max_height_vel = 0;
        max_height_accel = 0;

    case 3 % 
        enable = 1;
        height_ref = height_des;
        max_height_vel = fast_lim(1);
        max_height_accel = fast_lim(2);

    case 4
        enable = 1;
        height_ref = height_des;
        if (height_vel < 0)||(abs(height_cur - height_des) <= 0.1)||(height_des <= height_cur)
            max_height_vel = fast_lim(1);
            max_height_accel = fast_lim(2);
        else    
            max_height_vel = slow_lim(1);
            max_height_accel = slow_lim(2);
        end
    case 5
        enable = 1;
        height_ref = 0;
        if height_vel >= 0
            max_height_vel = fast_lim(1);
            max_height_accel = fast_lim(2);        
        else
            max_height_vel = slow_lim(1);
            max_height_accel = slow_lim(2);
        end
        
end

== matlab function Joystick_Visualization_2019a/Simple Drone Visualization/Pose Conditioning/Command Conditioning via Sigmoids/MATLAB Function4 ==
  data: sigmoid_type input; enable output; yaw_des input; slow_lim input; fast_lim input; yaw_cur input; yaw_ref output; max_yaw_vel output; max_yaw_accel output; yaw_vel input
function [enable, yaw_ref, max_yaw_vel, max_yaw_accel] = fcn(sigmoid_type, yaw_des, slow_lim, fast_lim, yaw_cur, yaw_vel)
%#codegen

enable = 0;
yaw_ref = 0;
max_yaw_vel = 0;
max_yaw_accel = 0;

switch sigmoid_type
    case 1 
        enable = 0;
        yaw_ref = 0;
        max_yaw_vel = 0;
        max_yaw_accel = 0;
    case 2
        enable = 1;
        yaw_ref = yaw_des;
        max_yaw_vel = slow_lim(1);
        max_yaw_accel = slow_lim(2);  
    case 3
        enable = 1;
        yaw_ref = yaw_des;
        max_yaw_vel = fast_lim(1);
        max_yaw_accel = fast_lim(2);
    case 4
        enable = 1;
        yaw_ref = yaw_des;
        if (yaw_vel < 0)||(yaw_des < yaw_cur)||(abs(yaw_cur-yaw_des)<=0.2)
            max_yaw_vel = fast_lim(1);
            max_yaw_accel = fast_lim(2);
        else    
            max_yaw_vel = slow_lim(1);
            max_yaw_accel = slow_lim(2);
        end
    case 5 
        enable = 1;
        yaw_ref = yaw_des;
        if (yaw_vel >= 0)
            max_yaw_vel = fast_lim(1);
            max_yaw_accel = fast_lim(2);
        else    
            max_yaw_vel = slow_lim(1);
            max_yaw_accel = slow_lim(2);
        end
end

== matlab function Joystick_Visualization_2019a/Simple Drone Visualization/Pose Conditioning/Command Conditioning via Sigmoids/Signmoid Type ==
  data: FSM_state input; sigmoid_type output
function sigmoid_type  = sigmoid_type_position(FSM_state)

% QDrone: Position Switchbox
%
% Logic for transforming/switching between available measurements as
% as well as commands depending on which state the FSM is in.
%
% v2.0 - 27th March, 2018
%
% INPUTS:
% -------
% FSM_state = current state of the FSM------------------------------------------------------- (#)         [1]
% 
% OUTPUTS:
% --------
% sigmoid = an integer whose state determines how the commands/measurements are transformed-- (#)         [1]

sigmoid_type = 0;

switch FSM_state
    case 1 % IDLE STATE
        sigmoid_type = 1;
    case 2 % ARM STATE
        sigmoid_type = 1;
    case 3 % TAKEOFF THROTTLE STATE
        sigmoid_type = 2;
    case 4 % TAKEOFF HEIGHT STATE
        sigmoid_type = 4;
    case 5 % FLIGHT STATE
        sigmoid_type = 3;
    case 6 % AUTOLAND STATE
        sigmoid_type = 5;
    case 7 % EMERGENCY STOP STATE
        sigmoid_type = 1;
    case 8 % EMERGENCY ABORT STATE
        sigmoid_type = 1;
    case 9 % DISABLE STATE
        sigmoid_type = 1;
end
